simulink model "nonlineardtm"  (R2018b)
settings: configuration reference "Physics" (kept outside this file)
model workspace (MAT data in the model file):
  x0_vehiclepose = Simulink.Parameter
  x0_vehiclepose.Value = [0 0 0]
  x0_vehiclepose.DataType = 'auto'
  x0_vehiclepose.Dimensions = [1 3]
undefined symbols (not defined in the file): Aerodynamics, Aligning, Antisway, Brakes, Compliance, ContactPatch, Environment, k1_TireFB_PT1, k1_WheelsFB_PT1, k2_TireFB_PT1, Kinematics, Lateral, Longitudinal, normalizeAngle, omega0_K_Vehicle_radps, omega0_Wheels_radps, Overturning, p_Tires_Pa, Rolling, Scaling, SensorData, Structural, TireSimulation, Turnslip, v0_K_Vehicle_mps, v0z_Wheels_mps, VehicleData, Vertical, Wheels, x0_verticaldynamics, z0_TireDeflection_m
libraries: vehdynlibtire x4, vehdynlibsuspension x2, vrlib x1, vehdynlibeom x1
(part 1 of 5)
settings Model: DataDictionary=nonlineardtm.sldd  ParameterArgumentNames=x0_vehiclepose  OrderedModelArguments=off  Creator=wischnewski  LastModifiedBy=ga76dol

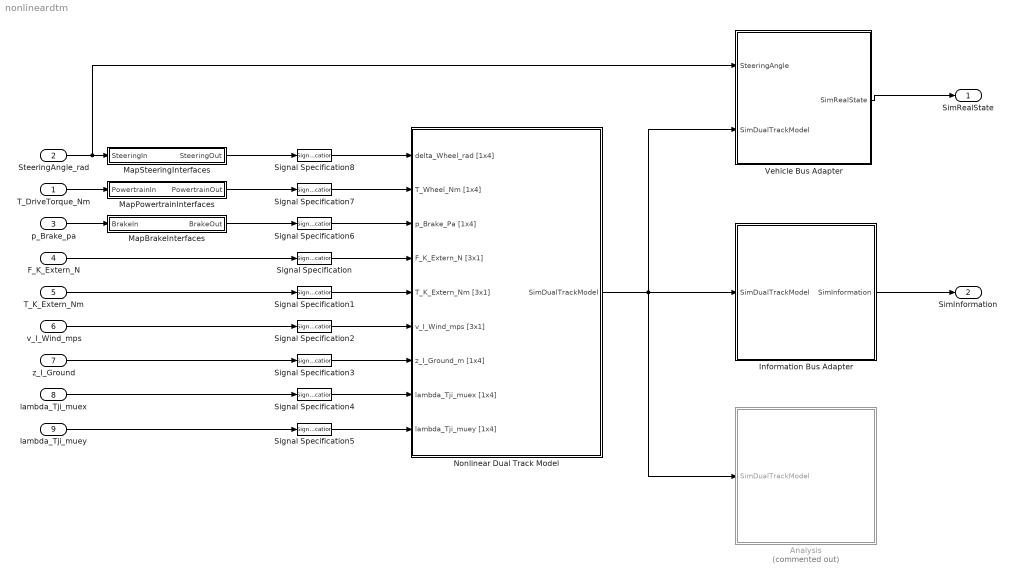
== system nonlineardtm ==
  T_DriveTorque_Nm : Inport  OutDataTypeStr=Bus: DriveTorque_Nm
  SteeringAngle_rad : Inport  Port=2
  p_Brake_pa : Inport  Port=3  OutDataTypeStr=Bus: BrakePressure_Pa
  F_K_Extern_N : Inport  Port=4
  T_K_Extern_Nm : Inport  Port=5
  v_I_Wind_mps : Inport  Port=6
  z_I_Ground : Inport  Port=7
  lambda_Tji_muex : Inport  Port=8
  lambda_Tji_muey : Inport  Port=9
  Analysis : Subsystem  Commented=on
  Information Bus Adapter : Subsystem
  MapBrakeInterfaces : Subsystem
  MapPowertrainInterfaces : Subsystem
  MapSteeringInterfaces : Subsystem
  Nonlinear Dual Track Model : Subsystem
  Signal Specification : SignalSpecification  Dimensions=[3,1]
  Signal Specification1 : SignalSpecification  Dimensions=[3,1]
  Signal Specification2 : SignalSpecification  Dimensions=[3,1]
  Signal Specification{3..8} (6 alike) : SignalSpecification  Dimensions=[1,4]
  Vehicle Bus Adapter : Subsystem
  SimRealState : Outport  OutDataTypeStr=Bus: SimRealState
  SimInformation : Outport  Port=2  OutDataTypeStr=Bus: SimInformation
  wires:
  T_K_Extern_Nm/1 -> Signal Specification1/1
  Vehicle Bus Adapter/1(SimRealState) -> SimRealState/1
  Nonlinear Dual Track Model/1(SimDualTrackModel) -> Vehicle Bus Adapter/2(SimDualTrackModel), Analysis/1(SimDualTrackModel), Information Bus Adapter/1(SimDualTrackModel)
  Information Bus Adapter/1(SimInformation) -> SimInformation/1
  lambda_Tji_muey/1 -> Signal Specification5/1
  lambda_Tji_muex/1 -> Signal Specification4/1
  z_I_Ground/1 -> Signal Specification3/1
  v_I_Wind_mps/1 -> Signal Specification2/1
  F_K_Extern_N/1 -> Signal Specification/1
  Signal Specification/1 -> Nonlinear Dual Track Model/4(F_K_Extern_N [3x1])
  Signal Specification1/1 -> Nonlinear Dual Track Model/5(T_K_Extern_Nm [3x1])
  Signal Specification2/1 -> Nonlinear Dual Track Model/6(v_I_Wind_mps [3x1])
  Signal Specification3/1 -> Nonlinear Dual Track Model/7(z_I_Ground_m [1x4])
  Signal Specification4/1 -> Nonlinear Dual Track Model/8(lambda_Tji_muex [1x4])
  Signal Specification5/1 -> Nonlinear Dual Track Model/9(lambda_Tji_muey [1x4])
  Signal Specification6/1 -> Nonlinear Dual Track Model/3(p_Brake_Pa [1x4])
  Signal Specification7/1 -> Nonlinear Dual Track Model/2(T_Wheel_Nm [1x4])
  Signal Specification8/1 -> Nonlinear Dual Track Model/1(delta_Wheel_rad [1x4])
  SteeringAngle_rad/1 -> Vehicle Bus Adapter/1(SteeringAngle), MapSteeringInterfaces/1(SteeringIn)
  MapSteeringInterfaces/1(SteeringOut) -> Signal Specification8/1
  T_DriveTorque_Nm/1 -> MapPowertrainInterfaces/1(PowertrainIn)
  MapPowertrainInterfaces/1(PowertrainOut) -> Signal Specification7/1
  p_Brake_pa/1 -> MapBrakeInterfaces/1(BrakeIn)
  MapBrakeInterfaces/1(BrakeOut) -> Signal Specification6/1

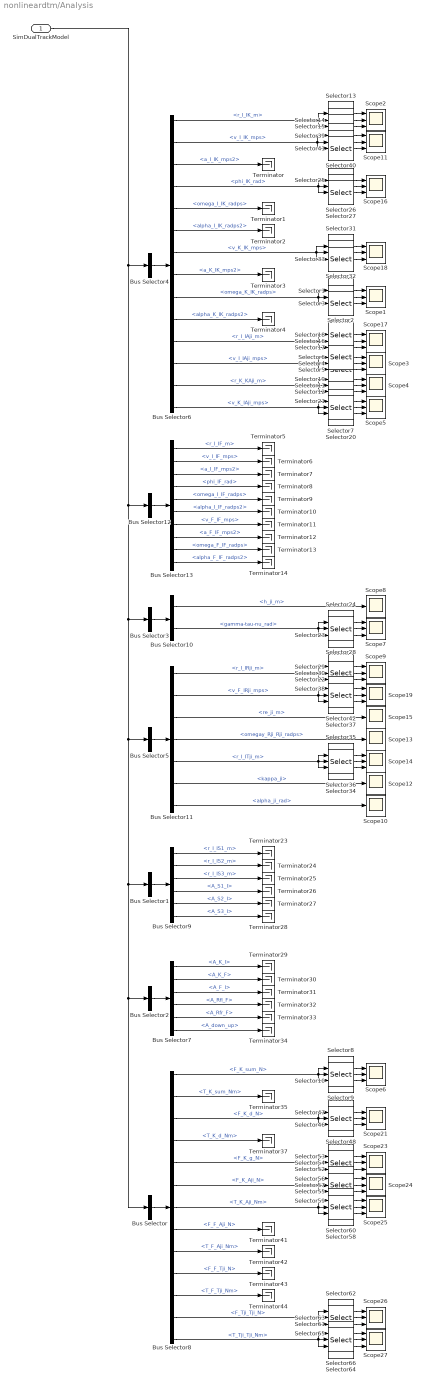
== system nonlineardtm/Analysis ==
  SimDualTrackModel : Inport
  Bus Selector : BusSelector  OutputSignals=SimForce  OutputAsBus=on
  Bus Selector1 : BusSelector  OutputSignals=SimSensor  OutputAsBus=on
  Bus Selector10 : BusSelector  OutputSignals=h_ji_m,gamma-tau-nu_rad
  Bus Selector11 : BusSelector  OutputSignals=r_I_IRji_m,v_F_IRji_mps,re_ji_m,omegay_Rji_Rji_radps,r_I_ITji_m,kappa_ji,alpha_ji_rad
  Bus Selector12 : BusSelector  OutputSignals=SimChassis  OutputAsBus=on
  Bus Selector13 : BusSelector  OutputSignals=r_I_IF_m,v_I_IF_mps,a_I_IF_mps2,phi_IF_rad,omega_I_IF_radps,alpha_I_IF_radps2,v_F_IF_mps,a_F_IF_mps2,omega_F_IF_radps,alpha_F_IF_radps2
  Bus Selector2 : BusSelector  OutputSignals=signal6  OutputAsBus=on
  Bus Selector3 : BusSelector  OutputSignals=SimSuspension  OutputAsBus=on
  Bus Selector4 : BusSelector  OutputSignals=signal1  OutputAsBus=on
  Bus Selector5 : BusSelector  OutputSignals=SimWheel  OutputAsBus=on
  Bus Selector6 : BusSelector  OutputSignals=r_I_IK_m,v_I_IK_mps,a_I_IK_mps2,phi_IK_rad,omega_I_IK_radps,alpha_I_IK_radps2,v_K_IK_mps,a_K_IK_mps2,omega_K_IK_radps,alpha_K_IK_radps2,r_I_IAji_m,v_I_IAji_mps,r_K_KAji_m,v_K_IAji_mps
  Bus Selector7 : BusSelector  OutputSignals=A_K_I,A_K_F,A_F_I,A_Rfl_F,A_Rfr_F,A_down_up
  Bus Selector8 : BusSelector  OutputSignals=F_K_sum_N,T_K_sum_Nm,F_K_d_N,T_K_d_Nm,F_K_g_N,F_K_Aji_N,T_K_Aji_Nm,F_F_Aji_N,T_F_Aji_Nm,F_F_Tji_N,T_F_Tji_Nm,F_Tji_Tji_N,T_Tji_Tji_Nm
  Bus Selector9 : BusSelector  OutputSignals=r_I_IS1_m,r_I_IS2_m,r_I_IS3_m,A_S1_I,A_S2_I,A_S3_I
  Scope{1..7,9,11,14,16..19,21,23..27} (20 alike) : Scope  NumInputPorts=3
  Scope{8,10,12..13,15} (5 alike) : Scope
  Selector{1,8,13,25,31,39,47,53} (8 alike) : Selector  InputPortWidth=3  IndexOptions=Index vector (dialog)  Indices=[1]  OutputSizes=1
  Selector{3,10,15,27,33,41,46,52} (8 alike) : Selector  InputPortWidth=3  IndexOptions=Index vector (dialog)  Indices=[3]  OutputSizes=1
  Selector{4,7,11,16,28,30,36,42,57,60,63,66} (12 alike) : Selector  NumberOfDimensions=2  InputPortWidth=3  IndexOptions=Index vector (dialog),Select all  Indices=2,1  OutputSizes=1,1
  Selector{5,12,17,20,22..23,34,37,55,58,61,64} (12 alike) : Selector  NumberOfDimensions=2  InputPortWidth=3  IndexOptions=Index vector (dialog),Select all  Indices=3,1  OutputSizes=1,1
  Selector{2,9,14,26,32,40,48,54} (8 alike) : Selector  InputPortWidth=3  IndexOptions=Index vector (dialog)  Indices=[2]  OutputSizes=1
  Selector{6,18..19,21,24,29,35,38,56,59,62,65} (12 alike) : Selector  NumberOfDimensions=2  InputPortWidth=3  IndexOptions=Index vector (dialog),Select all  Indices=1,1  OutputSizes=1,1
  Terminator{,1..14,23..35,37,41..44} (33 alike) : Terminator
  wires:
  SimDualTrackModel/1 -> Bus Selector12/1, Bus Selector5/1, Bus Selector/1, Bus Selector2/1, Bus Selector1/1, Bus Selector3/1, Bus Selector4/1
  Bus Selector12/1 -> Bus Selector13/1
  Bus Selector13/1 -> Terminator5/1  "<r_I_IF_m>"
  Bus Selector13/2 -> Terminator6/1  "<v_I_IF_mps>"
  Bus Selector13/3 -> Terminator7/1  "<a_I_IF_mps2>"
  Bus Selector13/4 -> Terminator8/1  "<phi_IF_rad>"
  Bus Selector13/5 -> Terminator9/1  "<omega_I_IF_radps>"
  Bus Selector13/6 -> Terminator10/1  "<alpha_I_IF_radps2>"
  Bus Selector13/7 -> Terminator11/1  "<v_F_IF_mps>"
  Bus Selector13/8 -> Terminator12/1  "<a_F_IF_mps2>"
  Bus Selector13/9 -> Terminator13/1  "<omega_F_IF_radps>"
  Bus Selector13/10 -> Terminator14/1  "<alpha_F_IF_radps2>"
  Bus Selector11/6 -> Scope12/1  "<kappa_ji>"
  Bus Selector11/7 -> Scope10/1  "<alpha_ji_rad>"
  Bus Selector11/4 -> Scope13/1  "<omegay_Rji_Rji_radps>"
  Bus Selector11/3 -> Scope15/1  "<re_ji_m>"
  Bus Selector11/1 -> Selector29/1, Selector30/1, Selector22/1  "<r_I_IRji_m>"
  Bus Selector5/1 -> Bus Selector11/1
  Bus Selector10/1 -> Scope8/1  "<h_ji_m>"
  Bus Selector3/1 -> Bus Selector10/1
  Bus Selector6/11 -> Selector16/1, Selector17/1, Selector18/1  "<r_I_IAji_m>"
  Bus Selector6/10 -> Terminator4/1  "<alpha_K_IK_radps2>"
  Bus Selector6/9 -> Selector2/1, Selector3/1, Selector1/1  "<omega_K_IK_radps>"
  Bus Selector6/8 -> Terminator3/1  "<a_K_IK_mps2>"
  Bus Selector6/7 -> Selector33/1, Selector32/1, Selector31/1  "<v_K_IK_mps>"
  Bus Selector6/6 -> Terminator2/1  "<alpha_I_IK_radps2>"
  Bus Selector6/5 -> Terminator1/1  "<omega_I_IK_radps>"
  Bus Selector6/4 -> Selector25/1, Selector27/1, Selector26/1  "<phi_IK_rad>"
  Bus Selector6/3 -> Terminator/1  "<a_I_IK_mps2>"
  Bus Selector6/2 -> Selector39/1, Selector41/1, Selector40/1  "<v_I_IK_mps>"
  Bus Selector6/1 -> Selector13/1, Selector15/1, Selector14/1  "<r_I_IK_m>"
  Bus Selector9/5 -> Terminator27/1  "<A_S2_I>"
  Bus Selector9/4 -> Terminator26/1  "<A_S1_I>"
  Bus Selector9/3 -> Terminator25/1  "<r_I_IS3_m>"
  Bus Selector9/2 -> Terminator24/1  "<r_I_IS2_m>"
  Bus Selector9/1 -> Terminator23/1  "<r_I_IS1_m>"
  Bus Selector9/6 -> Terminator28/1  "<A_S3_I>"
  Bus Selector1/1 -> Bus Selector9/1
  Bus Selector8/11 -> Terminator44/1  "<T_F_Tji_Nm>"
  Bus Selector8/10 -> Terminator43/1  "<F_F_Tji_N>"
  Bus Selector8/9 -> Terminator42/1  "<T_F_Aji_Nm>"
  Bus Selector8/8 -> Terminator41/1  "<F_F_Aji_N>"
  Bus Selector8/6 -> Selector57/1, Selector56/1, Selector55/1  "<F_K_Aji_N>"
  Bus Selector8/4 -> Terminator37/1  "<T_K_d_Nm>"
  Bus Selector8/2 -> Terminator35/1  "<T_K_sum_Nm>"
  Bus Selector/1 -> Bus Selector8/1
  Bus Selector7/6 -> Terminator34/1  "<A_down_up>"
  Bus Selector7/5 -> Terminator33/1  "<A_Rfr_F>"
  Bus Selector7/4 -> Terminator32/1  "<A_Rfl_F>"
  Bus Selector7/3 -> Terminator31/1  "<A_F_I>"
  Bus Selector7/2 -> Terminator30/1  "<A_K_F>"
  Bus Selector7/1 -> Terminator29/1  "<A_K_I>"
  Bus Selector2/1 -> Bus Selector7/1
  Bus Selector4/1 -> Bus Selector6/1
  Selector32/1 -> Scope18/2
  Selector40/1 -> Scope11/2
  Selector31/1 -> Scope18/1
  Selector13/1 -> Scope2/1
  Selector15/1 -> Scope2/3
  Selector26/1 -> Scope16/2
  Selector16/1 -> Scope17/2
  Selector27/1 -> Scope16/3
  Selector17/1 -> Scope17/3
  Selector33/1 -> Scope18/3
  Selector25/1 -> Scope16/1
  Selector18/1 -> Scope17/1
  Selector41/1 -> Scope11/3
  Selector39/1 -> Scope11/1
  Selector14/1 -> Scope2/2
  Selector1/1 -> Scope1/1
  Selector3/1 -> Scope1/3
  Selector2/1 -> Scope1/2
  Selector6/1 -> Scope3/1
  Selector5/1 -> Scope3/3
  Selector4/1 -> Scope3/2
  Bus Selector6/12 -> Selector6/1, Selector5/1, Selector4/1  "<v_I_IAji_mps>"
  Bus Selector6/13 -> Selector19/1, Selector11/1, Selector12/1  "<r_K_KAji_m>"
  Selector11/1 -> Scope4/2
  Selector12/1 -> Scope4/3
  Selector19/1 -> Scope4/1
  Selector21/1 -> Scope5/1
  Selector20/1 -> Scope5/3
  Selector7/1 -> Scope5/2
  Bus Selector6/14 -> Selector20/1, Selector7/1, Selector21/1  "<v_K_IAji_mps>"
  Selector9/1 -> Scope6/2
  Selector10/1 -> Scope6/3
  Selector8/1 -> Scope6/1
  Bus Selector8/1 -> Selector8/1, Selector9/1, Selector10/1  "<F_K_sum_N>"
  Bus Selector10/2 -> Selector23/1, Selector24/1, Selector28/1  "<gamma-tau-nu_rad>"
  Selector28/1 -> Scope7/2
  Selector23/1 -> Scope7/3
  Selector24/1 -> Scope7/1
  Selector29/1 -> Scope9/1
  Selector22/1 -> Scope9/3
  Selector30/1 -> Scope9/2
  Bus Selector11/5 -> Selector34/1, Selector35/1, Selector36/1  "<r_I_ITji_m>"
  Selector36/1 -> Scope14/2
  Selector34/1 -> Scope14/3
  Selector35/1 -> Scope14/1
  Bus Selector11/2 -> Selector37/1, Selector38/1, Selector42/1  "<v_F_IRji_mps>"
  Selector42/1 -> Scope19/2
  Selector37/1 -> Scope19/3
  Selector38/1 -> Scope19/1
  Bus Selector8/3 -> Selector47/1, Selector46/1, Selector48/1  "<F_K_d_N>"
  Selector47/1 -> Scope21/1
  Selector46/1 -> Scope21/3
  Selector48/1 -> Scope21/2
  Selector54/1 -> Scope23/2
  Selector52/1 -> Scope23/3
  Selector53/1 -> Scope23/1
  Bus Selector8/5 -> Selector54/1, Selector52/1, Selector53/1  "<F_K_g_N>"
  Selector56/1 -> Scope24/1
  Selector55/1 -> Scope24/3
  Selector57/1 -> Scope24/2
  Selector60/1 -> Scope25/2
  Selector58/1 -> Scope25/3
  Selector59/1 -> Scope25/1
  Bus Selector8/7 -> Selector58/1, Selector59/1, Selector60/1  "<T_K_Aji_Nm>"
  Bus Selector8/12 -> Selector63/1, Selector62/1, Selector61/1  "<F_Tji_Tji_N>"
  Selector62/1 -> Scope26/1
  Selector61/1 -> Scope26/3
  Selector63/1 -> Scope26/2
  Selector66/1 -> Scope27/2
  Selector64/1 -> Scope27/3
  Selector65/1 -> Scope27/1
  Bus Selector8/13 -> Selector64/1, Selector65/1, Selector66/1  "<T_Tji_Tji_Nm>"

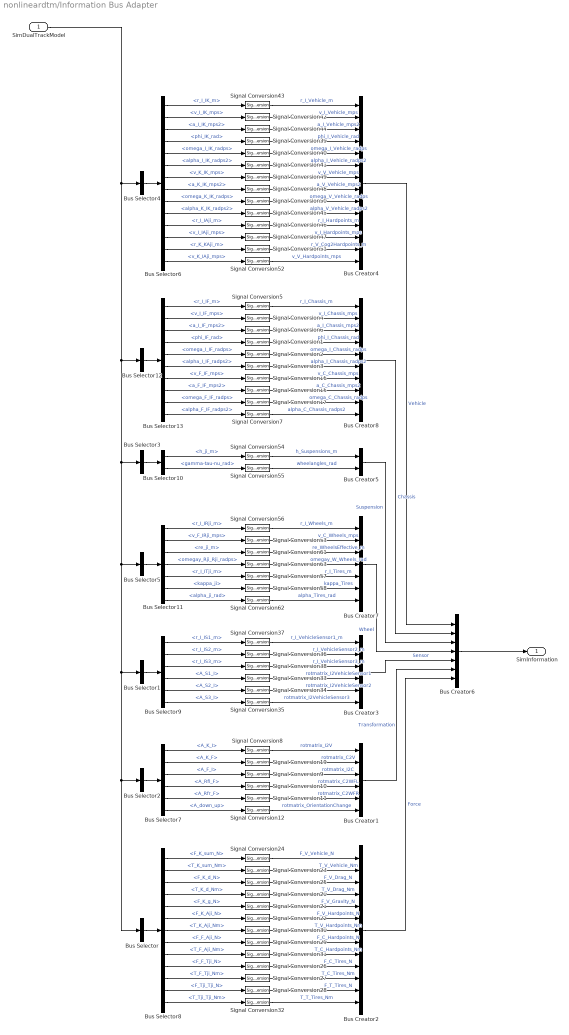
== system nonlineardtm/Information Bus Adapter ==
  SimDualTrackModel : Inport
  Bus Creator1 : BusCreator  Inputs=6  OutDataTypeStr=Bus: Transformation
      settings: InheritFromInputs=off
  Bus Creator2 : BusCreator  Inputs=13  OutDataTypeStr=Bus: Force
      settings: InheritFromInputs=off
  Bus Creator3 : BusCreator  Inputs=6  OutDataTypeStr=Bus: Sensor
      settings: InheritFromInputs=off
  Bus Creator4 : BusCreator  Inputs=14  OutDataTypeStr=Bus: Vehicle
      settings: InheritFromInputs=off
  Bus Creator5 : BusCreator  Inputs=2  OutDataTypeStr=Bus: Suspension
      settings: InheritFromInputs=off
  Bus Creator6 : BusCreator  Inputs=7  OutDataTypeStr=Bus: SimInformation
      settings: InheritFromInputs=off
  Bus Creator7 : BusCreator  Inputs=7  OutDataTypeStr=Bus: Wheel
      settings: InheritFromInputs=off
  Bus Creator8 : BusCreator  Inputs=10  OutDataTypeStr=Bus: Chassis
      settings: InheritFromInputs=off
  Bus Selector : BusSelector  OutputSignals=SimForce  OutputAsBus=on
  Bus Selector1 : BusSelector  OutputSignals=SimSensor  OutputAsBus=on
  Bus Selector10 : BusSelector  OutputSignals=h_ji_m,gamma-tau-nu_rad
  Bus Selector11 : BusSelector  OutputSignals=r_I_IRji_m,v_F_IRji_mps,re_ji_m,omegay_Rji_Rji_radps,r_I_ITji_m,kappa_ji,alpha_ji_rad
  Bus Selector12 : BusSelector  OutputSignals=SimChassis  OutputAsBus=on
  Bus Selector13 : BusSelector  OutputSignals=r_I_IF_m,v_I_IF_mps,a_I_IF_mps2,phi_IF_rad,omega_I_IF_radps,alpha_I_IF_radps2,v_F_IF_mps,a_F_IF_mps2,omega_F_IF_radps,alpha_F_IF_radps2
  Bus Selector2 : BusSelector  OutputSignals=signal6  OutputAsBus=on
  Bus Selector3 : BusSelector  OutputSignals=SimSuspension  OutputAsBus=on
  Bus Selector4 : BusSelector  OutputSignals=signal1  OutputAsBus=on
  Bus Selector5 : BusSelector  OutputSignals=SimWheel  OutputAsBus=on
  Bus Selector6 : BusSelector  OutputSignals=r_I_IK_m,v_I_IK_mps,a_I_IK_mps2,phi_IK_rad,omega_I_IK_radps,alpha_I_IK_radps2,v_K_IK_mps,a_K_IK_mps2,omega_K_IK_radps,alpha_K_IK_radps2,r_I_IAji_m,v_I_IAji_mps,r_K_KAji_m,v_K_IAji_mps
  Bus Selector7 : BusSelector  OutputSignals=A_K_I,A_K_F,A_F_I,A_Rfl_F,A_Rfr_F,A_down_up
  Bus Selector8 : BusSelector  OutputSignals=F_K_sum_N,T_K_sum_Nm,F_K_d_N,T_K_d_Nm,F_K_g_N,F_K_Aji_N,T_K_Aji_Nm,F_F_Aji_N,T_F_Aji_Nm,F_F_Tji_N,T_F_Tji_Nm,F_Tji_Tji_N,T_Tji_Tji_Nm
  Bus Selector9 : BusSelector  OutputSignals=r_I_IS1_m,r_I_IS2_m,r_I_IS3_m,A_S1_I,A_S2_I,A_S3_I
  Signal Conversion{1..12,15..17,19..58,61..63} (58 alike) : SignalConversion  OverrideOpt=off
  SimInformation : Outport  OutDataTypeStr=Bus: SimInformation
  wires:
  Bus Selector4/1 -> Bus Selector6/1
  Bus Selector2/1 -> Bus Selector7/1
  Bus Selector7/1 -> Signal Conversion8/1  "<A_K_I>"
  Bus Selector7/2 -> Signal Conversion19/1  "<A_K_F>"
  Bus Selector7/3 -> Signal Conversion9/1  "<A_F_I>"
  Bus Selector7/4 -> Signal Conversion10/1  "<A_Rfl_F>"
  Bus Selector7/5 -> Signal Conversion11/1  "<A_Rfr_F>"
  Bus Selector7/6 -> Signal Conversion12/1  "<A_down_up>"
  Signal Conversion8/1 -> Bus Creator1/1  "rotmatrix_I2V"
  Signal Conversion19/1 -> Bus Creator1/2  "rotmatrix_C2V"
  Signal Conversion9/1 -> Bus Creator1/3  "rotmatrix_I2C"
  Signal Conversion10/1 -> Bus Creator1/4  "rotmatrix_C2WFL"
  Signal Conversion11/1 -> Bus Creator1/5  "rotmatrix_C2WFR"
  Signal Conversion12/1 -> Bus Creator1/6  "rotmatrix_OrientationChange"
  Bus Selector/1 -> Bus Selector8/1
  Bus Selector8/1 -> Signal Conversion24/1  "<F_K_sum_N>"
  Bus Selector8/2 -> Signal Conversion23/1  "<T_K_sum_Nm>"
  Bus Selector8/3 -> Signal Conversion25/1  "<F_K_d_N>"
  Bus Selector8/4 -> Signal Conversion20/1  "<T_K_d_Nm>"
  Bus Selector8/5 -> Signal Conversion21/1  "<F_K_g_N>"
  Bus Selector8/6 -> Signal Conversion22/1  "<F_K_Aji_N>"
  Bus Selector8/7 -> Signal Conversion30/1  "<T_K_Aji_Nm>"
  Bus Selector8/8 -> Signal Conversion29/1  "<F_F_Aji_N>"
  Bus Selector8/9 -> Signal Conversion31/1  "<T_F_Aji_Nm>"
  Bus Selector8/10 -> Signal Conversion26/1  "<F_F_Tji_N>"
  Bus Selector8/11 -> Signal Conversion27/1  "<T_F_Tji_Nm>"
  Bus Selector8/12 -> Signal Conversion28/1  "<F_Tji_Tji_N>"
  Bus Selector8/13 -> Signal Conversion32/1  "<T_Tji_Tji_Nm>"
  Signal Conversion23/1 -> Bus Creator2/2  "T_V_Vehicle_Nm"
  Signal Conversion24/1 -> Bus Creator2/1  "F_V_Vehicle_N"
  Signal Conversion25/1 -> Bus Creator2/3  "F_V_Drag_N"
  Signal Conversion20/1 -> Bus Creator2/4  "T_V_Drag_Nm"
  Signal Conversion21/1 -> Bus Creator2/5  "F_V_Gravity_N"
  Signal Conversion22/1 -> Bus Creator2/6  "F_V_Hardpoints_N"
  Signal Conversion30/1 -> Bus Creator2/7  "T_V_Hardpoints_Nm"
  Signal Conversion29/1 -> Bus Creator2/8  "F_C_Hardpoints_N"
  Signal Conversion31/1 -> Bus Creator2/9  "T_C_Hardpoints_Nm"
  Signal Conversion26/1 -> Bus Creator2/10  "F_C_Tires_N"
  Signal Conversion27/1 -> Bus Creator2/11  "T_C_Tires_Nm"
  Signal Conversion28/1 -> Bus Creator2/12  "F_T_Tires_N"
  Signal Conversion32/1 -> Bus Creator2/13  "T_T_Tires_Nm"
  Bus Selector1/1 -> Bus Selector9/1
  Bus Selector9/6 -> Signal Conversion35/1  "<A_S3_I>"
  Signal Conversion35/1 -> Bus Creator3/6  "rotmatrix_I2VehicleSensor3"
  Bus Selector9/1 -> Signal Conversion37/1  "<r_I_IS1_m>"
  Bus Selector9/2 -> Signal Conversion36/1  "<r_I_IS2_m>"
  Bus Selector9/3 -> Signal Conversion38/1  "<r_I_IS3_m>"
  Bus Selector9/4 -> Signal Conversion33/1  "<A_S1_I>"
  Bus Selector9/5 -> Signal Conversion34/1  "<A_S2_I>"
  Signal Conversion36/1 -> Bus Creator3/2  "r_I_VehicleSensor2_m"
  Signal Conversion37/1 -> Bus Creator3/1  "r_I_VehicleSensor1_m"
  Signal Conversion38/1 -> Bus Creator3/3  "r_I_VehicleSensor3_m"
  Signal Conversion33/1 -> Bus Creator3/4  "rotmatrix_I2VehicleSensor1"
  Signal Conversion34/1 -> Bus Creator3/5  "rotmatrix_I2VehicleSensor2"
  Bus Selector6/1 -> Signal Conversion43/1  "<r_I_IK_m>"
  Bus Selector6/2 -> Signal Conversion42/1  "<v_I_IK_mps>"
  Bus Selector6/3 -> Signal Conversion44/1  "<a_I_IK_mps2>"
  Bus Selector6/4 -> Signal Conversion39/1  "<phi_IK_rad>"
  Bus Selector6/5 -> Signal Conversion40/1  "<omega_I_IK_radps>"
  Bus Selector6/6 -> Signal Conversion41/1  "<alpha_I_IK_radps2>"
  Bus Selector6/7 -> Signal Conversion49/1  "<v_K_IK_mps>"
  Bus Selector6/8 -> Signal Conversion48/1  "<a_K_IK_mps2>"
  Bus Selector6/9 -> Signal Conversion50/1  "<omega_K_IK_radps>"
  Bus Selector6/10 -> Signal Conversion45/1  "<alpha_K_IK_radps2>"
  Bus Selector6/11 -> Signal Conversion46/1  "<r_I_IAji_m>"
  Bus Selector6/12 -> Signal Conversion47/1  "<v_I_IAji_mps>"
  Bus Selector6/14 -> Signal Conversion52/1  "<v_K_IAji_mps>"
  Bus Selector6/13 -> Signal Conversion51/1  "<r_K_KAji_m>"
  Signal Conversion43/1 -> Bus Creator4/1  "r_I_Vehicle_m"
  Signal Conversion42/1 -> Bus Creator4/2  "v_I_Vehicle_mps"
  Signal Conversion44/1 -> Bus Creator4/3  "a_I_Vehicle_mps2"
  Signal Conversion39/1 -> Bus Creator4/4  "phi_I_Vehicle_rad"
  Signal Conversion40/1 -> Bus Creator4/5  "omega_I_Vehicle_radps"
  Signal Conversion41/1 -> Bus Creator4/6  "alpha_I_Vehicle_radps2"
  Signal Conversion49/1 -> Bus Creator4/7  "v_V_Vehicle_mps"
  Signal Conversion48/1 -> Bus Creator4/8  "a_V_Vehicle_mps2"
  Signal Conversion50/1 -> Bus Creator4/9  "omega_V_Vehicle_radps"
  Signal Conversion45/1 -> Bus Creator4/10  "alpha_V_Vehicle_radps2"
  Signal Conversion46/1 -> Bus Creator4/11  "r_I_Hardpoints_m"
  Signal Conversion47/1 -> Bus Creator4/12  "v_I_Hardpoints_mps"
  Signal Conversion51/1 -> Bus Creator4/13  "r_V_Cog2Hardpoints_m"
  Signal Conversion52/1 -> Bus Creator4/14  "v_V_Hardpoints_mps"
  Bus Selector3/1 -> Bus Selector10/1
  Signal Conversion55/1 -> Bus Creator5/2  "wheelangles_rad"
  Signal Conversion54/1 -> Bus Creator5/1  "h_Suspensions_m"
  Signal Conversion53/1 -> Bus Creator7/2  "v_C_Wheels_mps"
  Bus Selector10/1 -> Signal Conversion54/1  "<h_ji_m>"
  Bus Selector10/2 -> Signal Conversion55/1  "<gamma-tau-nu_rad>"
  Bus Selector11/2 -> Signal Conversion53/1  "<v_F_IRji_mps>"
  Bus Selector5/1 -> Bus Selector11/1
  Signal Conversion63/1 -> Bus Creator7/4  "omegay_W_Wheels_rad"
  Signal Conversion62/1 -> Bus Creator7/7  "alpha_Tires_rad"
  Signal Conversion58/1 -> Bus Creator7/6  "kappa_Tires"
  Signal Conversion57/1 -> Bus Creator7/5  "r_I_Tires_m"
  Signal Conversion56/1 -> Bus Creator7/1  "r_I_Wheels_m"
  Signal Conversion61/1 -> Bus Creator7/3  "re_WheelsEffective_m"
  Bus Selector11/1 -> Signal Conversion56/1  "<r_I_IRji_m>"
  Bus Selector11/3 -> Signal Conversion61/1  "<re_ji_m>"
  Bus Selector11/4 -> Signal Conversion63/1  "<omegay_Rji_Rji_radps>"
  Bus Selector11/7 -> Signal Conversion62/1  "<alpha_ji_rad>"
  Bus Selector11/6 -> Signal Conversion58/1  "<kappa_ji>"
  Bus Selector11/5 -> Signal Conversion57/1  "<r_I_ITji_m>"
  Bus Creator4/1 -> Bus Creator6/1  "Vehicle"
  Bus Creator7/1 -> Bus Creator6/4  "Wheel"
  Bus Creator3/1 -> Bus Creator6/5  "Sensor"
  Bus Creator1/1 -> Bus Creator6/6  "Transformation"
  Signal Conversion7/1 -> Bus Creator8/10  "alpha_C_Chassis_radps2"
  Signal Conversion17/1 -> Bus Creator8/9  "omega_C_Chassis_radps"
  Signal Conversion15/1 -> Bus Creator8/8  "a_C_Chassis_mps2"
  Signal Conversion16/1 -> Bus Creator8/7  "v_C_Chassis_mps"
  Signal Conversion3/1 -> Bus Creator8/6  "alpha_I_Chassis_radps2"
  Signal Conversion2/1 -> Bus Creator8/5  "omega_I_Chassis_radps"
  Signal Conversion1/1 -> Bus Creator8/4  "phi_I_Chassis_rad"
  Signal Conversion6/1 -> Bus Creator8/3  "a_I_Chassis_mps2"
  Signal Conversion4/1 -> Bus Creator8/2  "v_I_Chassis_mps"
  Signal Conversion5/1 -> Bus Creator8/1  "r_I_Chassis_m"
  Bus Selector13/10 -> Signal Conversion7/1  "<alpha_F_IF_radps2>"
  Bus Selector13/9 -> Signal Conversion17/1  "<omega_F_IF_radps>"
  Bus Selector13/8 -> Signal Conversion15/1  "<a_F_IF_mps2>"
  Bus Selector13/7 -> Signal Conversion16/1  "<v_F_IF_mps>"
  Bus Selector13/6 -> Signal Conversion3/1  "<alpha_I_IF_radps2>"
  Bus Selector13/5 -> Signal Conversion2/1  "<omega_I_IF_radps>"
  Bus Selector13/4 -> Signal Conversion1/1  "<phi_IF_rad>"
  Bus Selector13/3 -> Signal Conversion6/1  "<a_I_IF_mps2>"
  Bus Selector13/2 -> Signal Conversion4/1  "<v_I_IF_mps>"
  Bus Selector13/1 -> Signal Conversion5/1  "<r_I_IF_m>"
  Bus Selector12/1 -> Bus Selector13/1
  SimDualTrackModel/1 -> Bus Selector4/1, Bus Selector1/1, Bus Selector/1, Bus Selector2/1, Bus Selector5/1, Bus Selector3/1, Bus Selector12/1
  Bus Creator8/1 -> Bus Creator6/2  "Chassis"
  Bus Creator2/1 -> Bus Creator6/7  "Force"
  Bus Creator5/1 -> Bus Creator6/3  "Suspension"
  Bus Creator6/1 -> SimInformation/1

== system nonlineardtm/MapBrakeInterfaces ==
  BrakeIn : Inport
  Bus Selector : BusSelector  OutputSignals=p_BrakePressureFL_pa,p_BrakePressureFR_pa,p_BrakePressureRL_pa,p_BrakePressureRR_pa
  Matrix Concatenate1 : Concatenate  NumInputs=4  Mode=Multidimensional array  ConcatenateDimension=2
  Reshape : Reshape  OutputDimensionality=Row vector (2-D)
  BrakeOut : Outport
  wires:
  Matrix Concatenate1/1 -> Reshape/1
  BrakeIn/1 -> Bus Selector/1
  Reshape/1 -> BrakeOut/1
  Bus Selector/3 -> Matrix Concatenate1/3  "<p_BrakePressureRL_pa>"
  Bus Selector/4 -> Matrix Concatenate1/4  "<p_BrakePressureRR_pa>"
  Bus Selector/1 -> Matrix Concatenate1/1  "<p_BrakePressureFL_pa>"
  Bus Selector/2 -> Matrix Concatenate1/2  "<p_BrakePressureFR_pa>"

== system nonlineardtm/MapPowertrainInterfaces ==
  PowertrainIn : Inport
  Bus Selector : BusSelector  OutputSignals=T_DriveTorqueFL_Nm,T_DriveTorqueFR_Nm,T_DriveTorqueRL_Nm,T_DriveTorqueRR_Nm
  Matrix Concatenate : Concatenate  NumInputs=4  Mode=Multidimensional array  ConcatenateDimension=2
  Reshape : Reshape  OutputDimensionality=Row vector (2-D)
  PowertrainOut : Outport
  wires:
  PowertrainIn/1 -> Bus Selector/1
  Matrix Concatenate/1 -> Reshape/1
  Reshape/1 -> PowertrainOut/1
  Bus Selector/1 -> Matrix Concatenate/1  "<T_DriveTorqueFL_Nm>"
  Bus Selector/2 -> Matrix Concatenate/2  "<T_DriveTorqueFR_Nm>"
  Bus Selector/3 -> Matrix Concatenate/3  "<T_DriveTorqueRL_Nm>"
  Bus Selector/4 -> Matrix Concatenate/4  "<T_DriveTorqueRR_Nm>"

== system nonlineardtm/MapSteeringInterfaces ==
  SteeringIn : Inport  PortDimensions=1
  Constant : Constant  Value=0
  Gain : Gain  Gain=-1
  Matrix Concatenate : Concatenate  NumInputs=4  Mode=Multidimensional array  ConcatenateDimension=2
  Reshape : Reshape  OutputDimensionality=Row vector (2-D)
  SteeringOut : Outport
  wires:
  Reshape/1 -> SteeringOut/1
  Constant/1 -> Matrix Concatenate/4, Matrix Concatenate/3  "deltaR_rad"
  Matrix Concatenate/1 -> Reshape/1
  Gain/1 -> Matrix Concatenate/1, Matrix Concatenate/2
  SteeringIn/1 -> Gain/1
